simulink model "prob6_ad2"  (Simulink 7.8)
settings: Solver=ode45  StartTime=0.0  StopTime=4  RelTol=1e-3
values from neighbouring files (symbols this model uses):
  gamma = 0.1    [HW_4_6_setup.m]    (also in fitzhughnagumo2.m = 0.09)
settings Model: Creator=Dan  LastModifiedBy=Dan
settings DebuggingCC: FcnCallInpInsideContextMsg=Use local settings

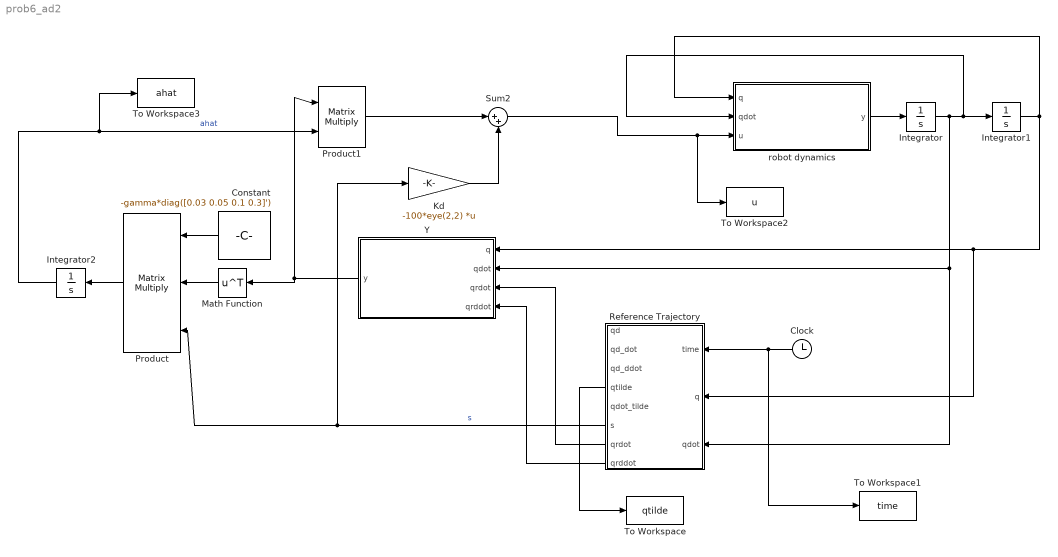
== system prob6_ad2 ==
  Clock : Clock
  Constant : Constant  Value=-gamma*diag([0.03 0.05 0.1 0.3]')
  Integrator : Integrator  InitialCondition=[0;0];
  Integrator1 : Integrator  InitialCondition=[0;0];
  Integrator2 : Integrator  InitialCondition=[0;0;0;0]'
  Kd : Gain  Gain=-100*eye(2,2)  Multiplication=Matrix(K*u)
  Math Function : Math  Operator=transpose  SaturateOnIntegerOverflow=on
  Product : Product  Inputs=3  Multiplication=Matrix(*)  RndMeth=Zero
  Product1 : Product  Multiplication=Matrix(*)  RndMeth=Zero
  Reference Trajectory : Subsystem
  Sum2 : Sum  Inputs=|++
  To Workspace : ToWorkspace  VariableName=qtilde  SampleTime=-1  SaveFormat=Array
  To Workspace1 : ToWorkspace  VariableName=time  SampleTime=-1  SaveFormat=Array
  To Workspace2 : ToWorkspace  VariableName=u  SampleTime=-1  SaveFormat=Array
  To Workspace3 : ToWorkspace  VariableName=ahat  SampleTime=-1  SaveFormat=Array
  Y : MATLAB Function  TreatAsAtomicUnit=on
  robot dynamics : MATLAB Function  TreatAsAtomicUnit=on
  wires:
  robot dynamics/1(y) -> Integrator/1
  Integrator/1 -> Integrator1/1, robot dynamics/2(qdot), Y/2(qdot), Reference Trajectory/3(qdot)
  Integrator1/1 -> Y/1(q), Reference Trajectory/2(q), robot dynamics/1(q)
  Clock/1 -> Reference Trajectory/1(time), To Workspace1/1
  Reference Trajectory/7(qrdot) -> Y/3(qrdot)
  Reference Trajectory/8(qrddot) -> Y/4(qrddot)
  Y/1(y) -> Math Function/1, Product1/1
  Constant/1 -> Product/1
  Math Function/1 -> Product/2
  Reference Trajectory/6(s) -> Product/3, Kd/1  "s"
  Product/1 -> Integrator2/1
  Integrator2/1 -> Product1/2, To Workspace3/1  "ahat"
  Product1/1 -> Sum2/1
  Kd/1 -> Sum2/2
  Sum2/1 -> robot dynamics/3(u), To Workspace2/1
  Reference Trajectory/4(qtilde) -> To Workspace/1

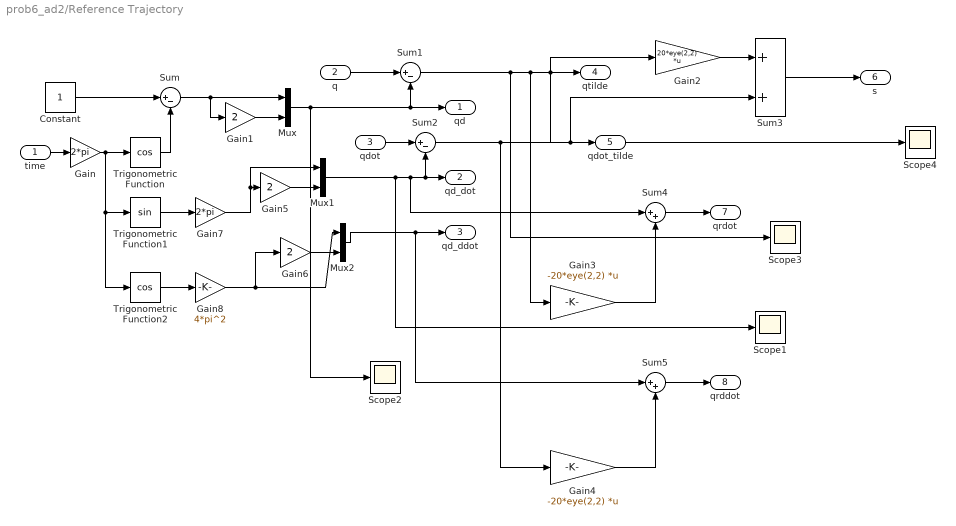
== system prob6_ad2/Reference Trajectory ==
  time : Inport
  q : Inport  Port=2
  qdot : Inport  Port=3
  Constant : Constant
  Gain : Gain  Gain=2*pi
  Gain1 : Gain  Gain=2
  Gain2 : Gain  Gain=20*eye(2,2)  Multiplication=Matrix(K*u)
  Gain3 : Gain  Gain=-20*eye(2,2)  Multiplication=Matrix(K*u)
  Gain4 : Gain  Gain=-20*eye(2,2)  Multiplication=Matrix(K*u)
  Gain5 : Gain  Gain=2
  Gain6 : Gain  Gain=2
  Gain7 : Gain  Gain=2*pi
  Gain8 : Gain  Gain=4*pi^2
  Mux : Mux  Inputs=2
  Mux1 : Mux  Inputs=2
  Mux2 : Mux  Inputs=2
  Scope{1..4} (4 alike) : Scope
      Scope1 settings: SaveName=ScopeData2
      Scope2 settings: SaveName=ScopeData4
      Scope3 settings: SaveName=ScopeData5
  Sum : Sum  Inputs=|+-
  Sum1 : Sum  Inputs=|+-
  Sum2 : Sum  Inputs=|+-
  Sum3 : Sum
  Sum4 : Sum  Inputs=|++
  Sum5 : Sum  Inputs=|++
  Trigonometric Function : Trigonometry  Operator=cos
  Trigonometric Function1 : Trigonometry
  Trigonometric Function2 : Trigonometry  Operator=cos
  qd : Outport
  qd_dot : Outport  Port=2
  qd_ddot : Outport  Port=3
  qtilde : Outport  Port=4
  qdot_tilde : Outport  Port=5
  s : Outport  Port=6
  qrdot : Outport  Port=7
  qrddot : Outport  Port=8
  wires:
  time/1 -> Gain/1
  Gain/1 -> Trigonometric Function/1, Trigonometric Function1/1, Trigonometric Function2/1
  Constant/1 -> Sum/1
  Trigonometric Function/1 -> Sum/2
  Sum/1 -> Mux/1, Gain1/1
  Gain1/1 -> Mux/2
  Mux/1 -> qd/1, Sum1/2, Scope2/1
  Mux1/1 -> qd_dot/1, Sum2/2, Sum4/1, Scope1/1
  Mux2/1 -> qd_ddot/1, Sum5/1
  q/1 -> Sum1/1
  Sum1/1 -> Gain2/1, qtilde/1, Scope4/1, Gain3/1, Scope3/1
  qdot/1 -> Sum2/1
  Sum2/1 -> qdot_tilde/1, Sum3/2, Gain4/1
  Gain2/1 -> Sum3/1
  Sum3/1 -> s/1
  Gain3/1 -> Sum4/2
  Sum4/1 -> qrdot/1
  Gain4/1 -> Sum5/2
  Sum5/1 -> qrddot/1
  Gain5/1 -> Mux1/2
  Trigonometric Function1/1 -> Gain7/1
  Gain7/1 -> Mux1/1, Gain5/1
  Trigonometric Function2/1 -> Gain8/1
  Gain8/1 -> Mux2/1, Gain6/1
  Gain6/1 -> Mux2/2

== matlab function Y ==
  data: q input double; y output double; qdot input double; qrdot input double; qrddot input double
function y = fcn(q,qdot,qrdot,qrddot)
%#codegen

y=zeros(2,4);

q1=q(1);
q2=q(2);
qdot1=qdot(1);
qdot2=qdot(2);

qrdot1=qrdot(1);
qrdot2=qrdot(2);
qrddot1=qrddot(1);
qrddot2=qrddot(2);

y(1,1)=qrddot1;
y(1,2)=qrddot2;
y(2,1)=0;
y(2,2)=qrddot1+qrddot2;
y(1,3)=(2*qrddot1+qrddot2)*cos(q2)-(qdot2*qrdot1+qdot1*qrdot2+qdot2*qrdot2)*sin(q2);
y(1,4)=(2*qrddot1+qrddot2)*sin(q2)+(qdot2*qrdot1+qdot1*qrdot2+qdot2*qrdot2)*cos(q2);
y(2,3)=qrddot1*cos(q2)+qdot1*qrdot1*sin(q2);
y(2,4)=qrddot1*sin(q2)-qdot1*qrdot1*cos(q2);

== matlab function robot dynamics ==
  data: q input double; y output double; qdot input double; u input double
function y = fcn(q,qdot,u)
%#codegen

q1=q(1);
q2=q(2);
qdot1=qdot(1);
qdot2=qdot(2);
g=9.81;

M1=1;
L1=1;
Me=2;
de=30*pi/180;
I1=0.12;
Lc1=0.5;
Ie=0.25;
Lce=0.6;

a1=I1+M1*Lc1^2+Ie+Me*Lce^2+Me*L1^2;
a2=Ie+Me*Lce^2;
a3=Me*L1*Lce*cos(de);
a4=Me*L1*Lce*sin(de);

H11=a1+2*a3*cos(q2)+2*a4*sin(q2);
H12=a2+a3*cos(q2)+a4*sin(q2);
H21=H12;
H22=a2;
h=a3*sin(q2)-a4*cos(q2);

G=[-M1*g*Lc1*cos(q1)-Me*g*L1*cos(q1)*Lce*cos(q1+q2);
    -Me*g*Lce*(cos(q1+q2))];

H=[H11 H12; H21 H22];
C=[-h*qdot2 -h*(qdot1+qdot2); h*qdot1 0];

y = -inv(H)*C*qdot+inv(H)*u;
